simulink model "FOC_physical_2_prototybe"  (R2024b)
settings: Solver=FixedStepAuto  StartTime=0.0  StopTime=3  FixedStep=1e-6  RelTol=1e-3
undefined symbols (not defined in the file): Down, GPTRIP1SEL, Ki_current, Ki_q, Ki_s, Ki_speed, Kp_current, Kp_q, Kp_s, Kp_speed, lambda, lamdaM, Ld, Ls, ma, P, Rs, T_max, T_period, Ts, TZ1, Up, Vdc
libraries: simulink x9, spsIGBTDiodeLib x6, spsCurrentMeasurementLib x3, eeStairGenerator x2, slpidlib x2, spsDCVoltageSourceLib x1, spsPermanentMagnetSynchronousMachineLib x1, c2802xlib x1, spsTriangleGeneratorLib x1, sps_lib x1
(part 2 of 2)

== system FOC_physical_2_prototybe/SVPWM1/Subsystem3 ==
  TS1 : Inport
  TS3 : Inport  Port=2
  TS5 : Inport  Port=3
  Carrier : Inport  Port=4
  Relational Operator : RelationalOperator  OutDataTypeStr=boolean  RndMeth=Simplest  InputSameDT=off
  Relational Operator1 : RelationalOperator  OutDataTypeStr=boolean  RndMeth=Simplest  InputSameDT=off
  Relational Operator2 : RelationalOperator  OutDataTypeStr=boolean  RndMeth=Simplest  InputSameDT=off
  Scope : Scope  NumInputPorts=3
  Pwm1 : Outport
  PWM3 : Outport  Port=2
  PWM5 : Outport  Port=3
  wires:
  Relational Operator2/1 -> PWM5/1
  Relational Operator1/1 -> PWM3/1
  Relational Operator/1 -> Pwm1/1, Scope/3
  Carrier/1 -> Relational Operator2/2, Relational Operator1/2, Relational Operator/2, Scope/2
  TS5/1 -> Relational Operator2/1
  TS3/1 -> Relational Operator1/1
  TS1/1 -> Relational Operator/1, Scope/1

== system FOC_physical_2_prototybe/SVPWM1/Subsystem4 ==
  TS1 : Inport
  TS3 : Inport  Port=2
  TS5 : Inport  Port=3
  NOT : Logic  Operator=NOT  IconShape=distinctive  AllPortsSameDT=off  OutDataTypeStr=boolean
  NOT1 : Logic  Operator=NOT  IconShape=distinctive  AllPortsSameDT=off  OutDataTypeStr=boolean
  NOT2 : Logic  Operator=NOT  IconShape=distinctive  AllPortsSameDT=off  OutDataTypeStr=boolean
  S1 : Outport
  S2 : Outport  Port=2
  S3 : Outport  Port=3
  S4 : Outport  Port=4
  S5 : Outport  Port=5
  S6 : Outport  Port=6
  wires:
  TS1/1 -> NOT/1, S1/1
  NOT/1 -> S4/1
  TS3/1 -> NOT1/1, S3/1
  NOT1/1 -> S6/1
  TS5/1 -> S5/1, NOT2/1
  NOT2/1 -> S2/1

== system FOC_physical_2_prototybe/SVPWM1/Valpha and Vbeta Clark Trans ==
  Va : Inport
  Vb : Inport  Port=2
  Vc : Inport  Port=3
  Add : Sum  Inputs=+++
  Add1 : Sum  Inputs=+-
  Gain : Gain  Gain=2/3
  Gain1 : Gain  Gain=-1/2
  Gain2 : Gain  Gain=-1/2
  Gain3 : Gain  Gain=2/3
  Gain5 : Gain  Gain=sqrt(3)/2
  Valpha : Outport
  Vbeta : Outport  Port=2
  wires:
  Gain5/1 -> Gain3/1
  Vc/1 -> Gain2/1, Add1/2
  Vb/1 -> Gain1/1, Add1/1
  Gain3/1 -> Vbeta/1
  Gain/1 -> Valpha/1
  Add/1 -> Gain/1
  Gain2/1 -> Add/3
  Add1/1 -> Gain5/1
  Va/1 -> Add/1
  Gain1/1 -> Add/2

== system FOC_physical_2_prototybe/Subsystem/Subsystem3 ==
  TS1 : Inport
  TS3 : Inport  Port=2
  TS5 : Inport  Port=3
  Carrier : Inport  Port=4
  Relational Operator : RelationalOperator  OutDataTypeStr=boolean  RndMeth=Simplest  InputSameDT=off
  Relational Operator1 : RelationalOperator  OutDataTypeStr=boolean  RndMeth=Simplest  InputSameDT=off
  Relational Operator2 : RelationalOperator  OutDataTypeStr=boolean  RndMeth=Simplest  InputSameDT=off
  Scope : Scope  NumInputPorts=3
  Pwm1 : Outport
  PWM3 : Outport  Port=2
  PWM5 : Outport  Port=3
  wires:
  Relational Operator2/1 -> PWM5/1
  Relational Operator1/1 -> PWM3/1
  Relational Operator/1 -> Pwm1/1, Scope/3
  Carrier/1 -> Relational Operator2/2, Relational Operator1/2, Relational Operator/2, Scope/2
  TS5/1 -> Relational Operator2/1
  TS3/1 -> Relational Operator1/1
  TS1/1 -> Relational Operator/1, Scope/1

== system FOC_physical_2_prototybe/Voltage limits/If Action Subsystem ==
  In3 : Inport
  In4 : Inport  Port=2
  Action Port : ActionPort  ActionPortLabel=if(u1 <= 0)
  Cast To Single : DataTypeConversion  OutDataTypeStr=single  SaturateOnIntegerOverflow=off  RndMeth=Floor
  Cast To Single1 : DataTypeConversion  OutDataTypeStr=single  SaturateOnIntegerOverflow=off  RndMeth=Floor
  Out2 : Outport
  Out3 : Outport  Port=2
  wires:
  In3/1 -> Cast To Single/1
  In4/1 -> Cast To Single1/1
  Cast To Single/1 -> Out2/1
  Cast To Single1/1 -> Out3/1

== system FOC_physical_2_prototybe/Voltage limits/If Action Subsystem1 ==
  In3 : Inport
  In4 : Inport  Port=2
  Action Port : ActionPort  ActionPortLabel=else
  Divide1 : Product  Inputs=*/  OutDataTypeStr=single
  Divide2 : Product  Inputs=/*  OutDataTypeStr=single
  Gain : Gain  Gain=sqrt(3)
  Gain1 : Gain  Gain=325 * .95
  Gain2 : Gain  Gain=325 * .95
  Square : Math  Operator=square  OutDataTypeStr=single
  Square Root : Sqrt  OutDataTypeStr=single  IntermediateResultsDataTypeStr=single
  Square1 : Math  Operator=square  OutDataTypeStr=single
  Sum : Sum  OutDataTypeStr=single  AccumDataTypeStr=single
  Out2 : Outport
  Out3 : Outport  Port=2
  wires:
  Divide1/1 -> Out2/1
  Divide2/1 -> Out3/1
  Square/1 -> Sum/1
  In3/1 -> Gain1/1, Square/1
  Sum/1 -> Square Root/1
  Gain2/1 -> Divide2/2
  Gain/1 -> Divide2/1, Divide1/2
  Gain1/1 -> Divide1/1
  Square1/1 -> Sum/2
  Square Root/1 -> Gain/1
  In4/1 -> Square1/1, Gain2/1

== system FOC_physical_2_prototybe/voltage limits by maintaining the same ration/Normal_Voltage ==
  Vq_ref_new : Inport
  Vd_ref_new : Inport  Port=2
  Action Port : ActionPort  ActionPortLabel=if(u1 <= 0)
  Data Type Conversion : DataTypeConversion  OutDataTypeStr=single  SaturateOnIntegerOverflow=off  RndMeth=Floor
  Data Type Conversion1 : DataTypeConversion  OutDataTypeStr=single  SaturateOnIntegerOverflow=off  RndMeth=Floor
  Vq_ref_1 : Outport
  Vd_ref_1 : Outport  Port=2
  wires:
  Vq_ref_new/1 -> Data Type Conversion/1
  Vd_ref_new/1 -> Data Type Conversion1/1
  Data Type Conversion/1 -> Vq_ref_1/1
  Data Type Conversion1/1 -> Vd_ref_1/1

== system FOC_physical_2_prototybe/voltage limits by maintaining the same ration/Voltage_to_be_Limited ==
  Vq_ref_new : Inport
  Vd_ref_new : Inport  Port=2
  Action Port : ActionPort  ActionPortLabel=else
  Divide1 : Product  Inputs=*/  OutDataTypeStr=single
  Divide2 : Product  Inputs=/*  OutDataTypeStr=single
  Gain : Gain  Gain=sqrt(3)
  Gain1 : Gain  Gain=Vdc * ma
  Gain2 : Gain  Gain=Vdc * ma
  Square : Math  Operator=square  OutDataTypeStr=single
  Square Root : Sqrt  OutDataTypeStr=single  IntermediateResultsDataTypeStr=single
  Square1 : Math  Operator=square  OutDataTypeStr=single
  Sum : Sum  OutDataTypeStr=single  AccumDataTypeStr=single
  Vq_ref_2 : Outport
  Vd_ref_2 : Outport  Port=2
  wires:
  Vq_ref_new/1 -> Gain1/1, Square/1
  Sum/1 -> Square Root/1
  Vd_ref_new/1 -> Square1/1, Gain2/1
  Square1/1 -> Sum/2
  Square/1 -> Sum/1
  Divide1/1 -> Vq_ref_2/1
  Square Root/1 -> Gain/1
  Divide2/1 -> Vd_ref_2/1
  Gain/1 -> Divide2/1, Divide1/2
  Gain1/1 -> Divide1/1
  Gain2/1 -> Divide2/2

== system FOC_physical_2_prototybe/SVPWM Technique/Step 1- Determine Vd, Vq, Vref, and angle/Polar form ==
  In1 : Inport
  In2 : Inport  Port=2
  Add : Sum
  Atan2 : Trigonometry  Operator=atan2
  Sqrt : Sqrt
  Square : Math  Operator=square
  Square1 : Math  Operator=square
  V ref : Outport
  angle : Outport  Port=2
  wires:
  In1/1 -> Square/1, Atan2/2
  Add/1 -> Sqrt/1
  Sqrt/1 -> V ref/1
  In2/1 -> Square1/1, Atan2/1
  Atan2/1 -> angle/1
  Square/1 -> Add/1
  Square1/1 -> Add/2

== system FOC_physical_2_prototybe/SVPWM Technique/Step 1- Determine Vd, Vq, Vref, and angle/Power variant Clark transformation  ==
  Va : Inport
  Vb : Inport  Port=2
  Vc : Inport  Port=3
  Gain : Gain  Gain=0.5
  Gain1 : Gain  Gain=0.5
  Gain2 : Gain  Gain=2/3
  Gain3 : Gain  Gain=sqrt(3)/2
  Gain4 : Gain  Gain=2/3
  Sum : Sum  Inputs=+--
  Sum1 : Sum  Inputs=+-
  V alpha : Outport
  V beta : Outport  Port=2
  wires:
  Gain4/1 -> V beta/1
  Gain2/1 -> V alpha/1
  Vb/1 -> Gain/1, Sum1/1
  Gain/1 -> Sum/2
  Sum1/1 -> Gain3/1
  Gain1/1 -> Sum/3
  Vc/1 -> Gain1/1, Sum1/2
  Sum/1 -> Gain2/1
  Gain3/1 -> Gain4/1
  Va/1 -> Sum/1

== system FOC_physical_2_prototybe/SVPWM Technique/Step 2- Determine time duration T1, T2, T/angle_d ==
  angle : Inport
  Sector : Inport  Port=2
  Constant3 : Constant
  Gain : Gain  Gain=pi/3
  Subtract4 : Sum  Inputs=-+
  Subtract5 : Sum  Inputs=+-
  angle_d(0 - pi/3) : Outport
  wires:
  Gain/1 -> Subtract4/1
  Subtract5/1 -> Gain/1
  Constant3/1 -> Subtract5/2
  Subtract4/1 -> angle_d(0 - pi/3)/1
  Sector/1 -> Subtract5/1
  angle/1 -> Subtract4/2

== system FOC_physical_2_prototybe/SVPWM1/Subsystem1/Theta dash ==
  Sector : Inport
  angle : Inport  Port=2
  Constant : Constant
  Display : Display
  Gain : Gain  Gain=(pi/3)
  Subtract : Sum  Inputs=-+
  Subtract1 : Sum  Inputs=-+
  Theta dash : Outport
  wires:
  Subtract/1 -> Theta dash/1, Display/1
  Subtract1/1 -> Gain/1
  Sector/1 -> Subtract1/2
  Constant/1 -> Subtract1/1
  Gain/1 -> Subtract/1
  angle/1 -> Subtract/2

== matlab function FOC_physical_2_prototybe/SVPWM Technique/Sector Detector ==
  data: u input; S output
function S = fcn(u)

  u= 180/(pi)*u ; % rad to degree
  
if (u>=0)&&(u<60)
  u = 1  ; 
elseif (u>=60)&&(u<120)
  u = 2  ;  
elseif (u>=120)&&(u<180)
  u = 3  ;  
elseif (u>=-180)&&(u<-120)
  u = 4  ;
elseif (u>=-120)&&(u<-60)
  u = 5  ;
elseif (u>=-60)&&(u<0)
  u = 6  ;
else
  u=0 ; 
end

S = u;

== matlab function FOC_physical_2_prototybe/SVPWM Technique/Step 3- Determine the switching time of each transistor (S1 to S6) /Sector detection1 ==
  data: s input; u input; Ts1 output; Ts3 output; v input; w input; g input; Ts5 output
function [Ts1,Ts3,Ts5] = fcn(s,u,v,w,g)

switch s 
  
 case 1 
  Ts1 = u ; 
  Ts3 = v ;
  Ts5 = w ;
 case 2 
  Ts1 = g ; 
  Ts3 = u ; 
  Ts5 = w ;
 case 3 
  Ts1 = w ;
  Ts3 = u ; 
  Ts5 = v ; 
 case 4 
  Ts1 = w ;
  Ts3 = g ; 
  Ts5 = u ;
 case 5 
  Ts1 = v ;
  Ts3 = w ; 
  Ts5 = u ;
 case 6 
  Ts1 = u ;
  Ts3 = w ; 
  Ts5 = g ;
 otherwise 
 Ts1 = 0 ; 
 Ts3 = 0 ;
 Ts5 = 0 ;
 end 

end

== matlab function FOC_physical_2_prototybe/MATLAB Function ==
  settings: updateMethod=DISCRETE
  data: omega_est output; v_alpha input; theta_est output; v_beta input; i_alpha input; i_beta input; Ts input; reset input
function [omega_est, theta_est] = ekf_pmsm_simplified_ab(v_alpha, v_beta, i_alpha, i_beta, Ts, reset)
% EKF_PMSM_SIMPLIFIED_AB  Simplified EKF for PMSM sensorless control.
%
%   [omega_est, theta_est] = EKF_PMSM_SIMPLIFIED_AB(v_alpha, v_beta, i_alpha, i_beta, Ts)
%   estimates the electrical rotor speed (rad/s) and angle (rad) using the
%   steady‑state d‑q model (Section III, Tondpoor et al. 2020). The inputs
%   are voltages and currents in the stationary α‑β frame.
%
%   Inputs:
%       v_alpha, v_beta  – stator voltages (α‑β) [V] (e.g. reference voltages)
%       i_alpha, i_beta  – measured stator currents (α‑β) [A]
%       Ts               – sampling time [s] (used for angle integration)
%       reset            – (optional) true to reinitialize the filter
%                           (call once before starting a new run)
%
%   Outputs:
%       omega_est   – estimated electrical angular velocity [rad/s]
%       theta_est   – estimated electrical angle [rad] (0 to 2*pi)
%
%   The filter uses a persistent state vector [v_d; v_q; omega_e] and the
%   corresponding covariance matrix.  Angles are integrated outside the EKF
%   recursion and fed back to perform the Park transformation.
%
%   Example:
%       % Initialisation call
%       [w, th] = ekf_pmsm_simplified_ab(valpha, vbeta, ialpha, ibeta, 100e-6, true);
%       % Loop
%       for k = 1:...
%           [w, th] = ekf_pmsm_simplified_ab(valpha, vbeta, ialpha, ibeta, 100e-6);
%           % ... use w, th for field-oriented control ...
%       end

%#codegen   % compatible with automatic C code generation

% --- Motor Parameters (tune to your PMSM) ---
R       = 1.45;      % phase resistance [Ohm]
L       = 6.2e-3;   % phase inductance (surface‑mounted: Ld = Lq) [H]
psi_pm  = 0.062;    % permanent‑magnet flux linkage [Wb]

% --- EKF Noise Covariances (tune for your application) ---
% Process noise: Q = diag([Q_vd, Q_vq, Q_w])
Q_vd    = 0.01;     % d‑axis voltage uncertainty
Q_vq    = 0.01;     % q‑axis voltage uncertainty
Q_w     = 100;      % speed uncertainty (rad/s)^2 – higher = faster tracking
Q       = diag([Q_vd, Q_vq, Q_w]);

% Measurement noise: R = diag([R_vd, R_vq])
R_vd    = 0.1;      % voltage measurement noise (d‑axis)
R_vq    = 0.1;      % voltage measurement noise (q‑axis)
R_meas  = diag([R_vd, R_vq]);

% --- Persistent states (preserve between calls) ---
persistent x_hat P_hat theta_prev

% --- Initialisation (on first call or explicit reset) ---
if isempty(x_hat) || (nargin >= 6 && reset)
    % Initial guess: zero voltages, zero speed
    x_hat   = [0; 0; 0];          % [v_d_est; v_q_est; omega_est]
    P_hat   = diag([1, 1, 10]);   % initial covariance
    theta_prev = 0;               % initial angle (will be updated after first integration)
end

% --- 1) Park transformation using the previous angle estimate ---
%    (this gives d‑q currents and voltages as seen by the previous frame)
c = cos(theta_prev);
s = sin(theta_prev);

i_d =  c * i_alpha + s * i_beta;
i_q = -s * i_alpha + c * i_beta;

v_d_meas =  c * v_alpha + s * v_beta;
v_q_meas = -s * v_alpha + c * v_beta;

% --- 2) EKF prediction step (state: x = [v_d; v_q; omega_e]) ---
% The system model:  v_d = R*i_d - L*omega_e*i_q
%                     v_q = R*i_q + (L*i_d + psi_pm)*omega_e
%                     omega_e = omega_e  (assumed constant within one sample)
%
% Here the “input” is the measured d‑q currents, used in the prediction of
% the d‑q voltages.  The state prediction uses the *current* samples of
% i_d, i_q (not previous ones, to avoid one‑step lag).

omega_prev = x_hat(3);

% State update: x_k^- = f( x_{k-1}^+, u_k )
% With u_k = [i_d; i_q] (from the current sample)
x_minus = [ R*i_d - L*omega_prev*i_q;
            R*i_q + (L*i_d + psi_pm)*omega_prev;
            omega_prev ];

% Jacobian F = df/dx evaluated at (x_{k-1}^+, u_k)
F13 = -L * i_q;
F23 =  L * i_d + psi_pm;

% Efficient covariance prediction (Eq. (18) in the paper)
% Only element P33 is propagated into the larger matrix.
P33 = P_hat(3,3);
P_minus = zeros(3);
P_minus(1,1) = P33 * F13^2 + Q_vd;
P_minus(2,2) = P33 * F23^2 + Q_vq;
P_minus(3,3) = P33 + Q_w;
P_minus(1,2) = P33 * F13 * F23;
P_minus(2,1) = P_minus(1,2);
P_minus(1,3) = P33 * F13;
P_minus(3,1) = P_minus(1,3);
P_minus(2,3) = P33 * F23;
P_minus(3,2) = P_minus(2,3);

% --- 3) EKF update (measurement: y = [v_d_meas; v_q_meas]) ---
H = [1, 0, 0;  0, 1, 0];      % output matrix: y = [x1; x2]
y_pred = x_minus(1:2);
innov  = [v_d_meas; v_q_meas] - y_pred;

S = H * P_minus * H' + R_meas;   % innovation covariance
K = P_minus * H' / S;            % Kalman gain (matrix right‑division)

x_hat = x_minus + K * innov;
P_hat = (eye(3) - K * H) * P_minus;

% --- 4) Integrate estimated speed to obtain the new angle ---
theta_est = theta_prev + x_hat(3) * Ts;
theta_est = mod(theta_est, 2*pi);   % wrap to [0, 2*pi)

% --- 5) Store the new angle and outputs ---
theta_prev = theta_est;          % update for next call
omega_est  = x_hat(3);           % estimated electrical speed

end

== matlab function FOC_physical_2_prototybe/MATLAB Function1 ==
  settings: updateMethod=DISCRETE
  data: omega_mech output; vd_meas input; theta_mech output; vq_meas input; id input; iq input; Ts input
function [omega_mech, theta_mech] = ekf_simplified_paper_aligned(vd_meas, vq_meas, id, iq, Ts)
% ekf_simplified_paper_aligned
% Simplified EKF + angle correction loop → the estimated angle will
% synchronise with the rotor even if the speed estimate has a small bias.
%
% Inputs:  vd_meas, vq_meas – measured d‑q voltages
%          id, iq – measured d‑q currents
%          Ts – sampling time [s]
% Outputs:
%   omega_mech : estimated mechanical speed [rad/s]
%   theta_mech : estimated mechanical angle [rad] (0 … 2π), aligned to rotor

% ------------------- MOTOR PARAMETERS (Y-2012-2) -------------------------
R     = 1.45;       % stator phase resistance [Ohm]
L     = 6.2e-3;     % stator inductance [H]
psi_f = 0.062;       % PM flux linkage [Wb]   (from Kt = 0.37 Nm/A, 8 poles)
p     = 4;           % pole pairs
% -------------------------------------------------------------------------

% --------- TUNED NOISE COVARIANCES (keep fast convergence) ----------------
Q     = diag([0.01, 0.01, 800]);   % process noise
R_kal = 0.1 * eye(2);              % measurement noise
P0_speed = 2000;                   % initial speed uncertainty
% -------------------------------------------------------------------------

% --------- ANGLE CORRECTION GAIN (tune this value) ------------------------
% Start with 0.2; increase if angle converges too slowly, decrease if it oscillates.
K_angle = 0.2;     % electrical rad per (V·s)  -- the sign may need to be flipped
% -------------------------------------------------------------------------

persistent x_hat Pmat theta_elec_corr_prev initialized
persistent theta_mech_raw_prev

if isempty(initialized)
    x_hat = [vd_meas; vq_meas; 0];          % [v_d; v_q; ω_e]
    Pmat  = diag([10, 10, P0_speed]);
    theta_elec_corr_prev = 0;               % corrected electrical angle
    theta_mech_raw_prev = 0;
    initialized = true;
end

%% ================== EKF Prediction Step =================================
omega_elec_prev = x_hat(3);

x_pred = [ R*id - L*omega_elec_prev*iq;
           R*iq + (L*id + psi_f)*omega_elec_prev;
           omega_elec_prev ];

F13 = -L * iq;
F23 =  L * id + psi_f;
F = [0, 0, F13;
     0, 0, F23;
     0, 0, 1];

P_pred = F * Pmat * F' + Q;
P_pred = (P_pred + P_pred') / 2;

%% ================== EKF Update Step =====================================
y_est = x_pred(1:2);
y_meas = [vd_meas; vq_meas];
innovation = y_meas - y_est;          % [v_d_err; v_q_err]
H = [1, 0, 0;
     0, 1, 0];
S = H * P_pred * H' + R_kal;
K = P_pred * H' / S;
x_hat = x_pred + K * innovation;
Pmat = (eye(3) - K * H) * P_pred;
Pmat = (Pmat + Pmat') / 2;

% Estimated electrical speed from EKF
omega_elec = x_hat(3);

%% ================== Angle correction loop ===============================
% Pure integration of speed
theta_elec_open = theta_elec_corr_prev + Ts * omega_elec;

% Correction term from d‑axis voltage error:
%   If the estimated angle is lagging, v_d_meas will contain a projection
%   of the actual back‑EMF (which should appear only on q‑axis for a
%   correctly aligned frame).  The sign of K_angle must be chosen such that
%   this term drives the angle error to zero.
correction = K_angle * innovation(1);   % innovation(1) = v_d_meas - v_d_est

theta_elec_corr = theta_elec_open + Ts * correction;   % corrected electrical angle

% Store for next iteration
theta_elec_corr_prev = theta_elec_corr;

%% ================== Mechanical outputs ==================================
% Unwrapped raw mechanical angle for spike‑free speed computation
theta_mech_raw = theta_elec_corr / p;
omega_mech = (theta_mech_raw - theta_mech_raw_prev) / Ts;
theta_mech_corr = mod(theta_mech_raw, 2*pi);   % wrapped for output

theta_mech_raw_prev = theta_mech_raw;

theta_mech = theta_mech_corr;   % final aligned angle
omega_mech = omega_mech;        % speed
end

== matlab function FOC_physical_2_prototybe/MATLAB Function2 ==
  settings: updateMethod=DISCRETE
  data: omega_est_mech output; vd input; theta_est_elec output; vq input; id input; iq input; Ts input
function [omega_est_mech, theta_est_elec] = ekf_simplified(vd, vq, id, iq, Ts)
    % SIMPLIFIED EKF (Tondpoor et al. 2020)
    
    % =====================================================================
    % 1. MOTOR PARAMETERS
    % =====================================================================
    r      = 1.45;       % Phase resistance [Ohm]
    L      = 6.2e-3;     % Phase inductance [H] (Use Lq if IPMSM)
    psi_pm = 0.062;      % PM flux linkage [Wb]
    p      = 4;          % Pole Pairs

    % 2. Persistent Variables
    persistent x_hat P theta omega_filtered
    if isempty(x_hat)
        x_hat = zeros(3,1); 
        P = eye(3) * 0.1;
        theta = 0; 
        omega_filtered = 0;
    end

    % 3. Covariance Matrices
    Q = diag([1.0, 1.0, 50.0]); 
    R = diag([1.0, 1.0]);       

    % Inputs
    u_id = id;
    u_iq = iq;
    y = [vd; vq]; % MUST BE IN TRUE VOLTS!

    we_h = x_hat(3);

    % =====================================================================
    % PREDICTION
    % =====================================================================
    x_minus = zeros(3,1);
    x_minus(1) = r*u_id - L*we_h*u_iq;
    x_minus(2) = r*u_iq + (L*u_id + psi_pm)*we_h;
    x_minus(3) = we_h;

    F13 = -L*u_iq;
    F23 = L*u_id + psi_pm;
    
    P33 = P(3,3);
    P_minus = zeros(3,3);
    P_minus(1,1) = P33*(F13^2) + Q(1,1);
    P_minus(1,2) = F13*F23*P33;
    P_minus(1,3) = F13*P33;
    P_minus(2,1) = P_minus(1,2);
    P_minus(2,2) = P33*(F23^2) + Q(2,2);
    P_minus(2,3) = F23*P33;
    P_minus(3,1) = P_minus(1,3);
    P_minus(3,2) = P_minus(2,3);
    P_minus(3,3) = P33 + Q(3,3);

    % =====================================================================
    % UPDATE
    % =====================================================================
    H = [1, 0, 0;
         0, 1, 0];

    S = H * P_minus * H' + R;
    K = P_minus * H' / S;

    innovation = y - H * x_minus;
    x_hat = x_minus + K * innovation;
    P = (eye(3) - K * H) * P_minus;

    % =====================================================================
    % OUTPUTS
    % =====================================================================
    omega_est_elec = x_hat(3);
    
    % Low pass filter to smooth the speed scope output (Optional but helpful)
    % Alpha = Ts / (Ts + tau), assuming Ts=1e-5 and tau=0.001
    alpha = 0.01; 
    omega_filtered = (1 - alpha) * omega_filtered + alpha * omega_est_elec;
    
    % OUTPUT 1: Mechanical Speed for the Scope (rad/s)
    % Multiply by (60/(2*pi)) outside the block if you want RPM
    omega_est_mech = omega_filtered / p; 
    
    % Integrate Electrical Speed to get Electrical Angle
    theta = theta + omega_est_elec * Ts;
    
    if theta > 2*pi
        theta = theta - 2*pi;
    elseif theta < 0
        theta = theta + 2*pi;
    end
    
    % OUTPUT 2: Electrical Angle (Feed this directly to Park transforms!)
    theta_est_elec = theta;
end

== matlab function FOC_physical_2_prototybe/SVPWM1/Sector detection ==
  data: u input; S output
function S = fcn(u)

u = (180/pi)* u;

if(u < 60 && u >= 0)
    u = 1;
elseif(u < 120 && u >= 60)
    u = 2;
elseif(u < 180 && u >= 120)
    u = 3;
elseif(u < -120 && u >= -180)
u = 4;
elseif(u < -60 && u >= -120)
u = 5;
elseif(u < 0 && u >= -60)
u = 6;
else
    u = 0;
end
S = u;

== matlab function FOC_physical_2_prototybe/SVPWM1/Subsystem2/MATLAB Function ==
  data: TS1 output; u input; TS3 output; TS5 output; v input; w input; g input; S input
function [TS1, TS3,TS5] = fcn(u, v, w, g,S)

switch S
    case 1
        TS1 = u;
        TS3 = v;
        TS5 = w;
    case 2
        TS1 = g;
        TS3 = u;
        TS5 = w;
    case 3
        TS1 = w;
        TS3 = u;
        TS5 = v;
    case 4
        TS1 = w;
        TS3 = g;
        TS5 = u;
    case 5
        TS1 = v;
        TS3 = w;
        TS5 = u;
    case 6
        TS1 = u;
        TS3 = w;
        TS5 = g;
    otherwise
      TS1=0;  
      TS3=0;  
      TS5=0; 
end
end
